simulink model "sldemo_tc_blocks"  (Simulink 7.6)
settings: Solver=FixedStepDiscrete  StartTime=0.0  StopTime=1  FixedStep=1  RelTol=1e-3
model workspace: external: MAT-File sldemo_tc_blocks_data.mat (data not in the file)
values from neighbouring files (symbols this model uses):
  TypeB_degC = TypeB_degC(1:2:end)    [sldemo_create_tc_blocks_data.m]    (also in sldemo_tc_blocks_data.mat = [0 2 4 6 8 10 12 14 16 18 20 22 ... (911 elements, 1x911)])
  TypeB_Volts = tcvoltage('B', TypeB_degC)    [sldemo_create_tc_blocks_data.m]    (also in sldemo_tc_blocks_data.mat = [0 -4.69410779782e-07 -8.91652511353e-07 -1.2667879384e-06 -)
  TypeE_degC = TypeE_degC(1:2:end)    [sldemo_create_tc_blocks_data.m]    (also in sldemo_tc_blocks_data.mat = [-270 -268 -266 -264 -262 -260 -258 -256 -254 -252 -250 -248)
  TypeE_Volts = tcvoltage('E', TypeE_degC)    [sldemo_create_tc_blocks_data.m]    (also in sldemo_tc_blocks_data.mat = [-0.00983495085619 -0.00983083480791 -0.00982483890705 -0.00)
  TypeJ_degC = TypeJ_degC(1:2:end)    [sldemo_create_tc_blocks_data.m]    (also in sldemo_tc_blocks_data.mat = [-210 -208 -206 -204 -202 -200 -198 -196 -194 -192 -190 -188)
  TypeJ_Volts = tcvoltage('J', TypeJ_degC)    [sldemo_create_tc_blocks_data.m]    (also in sldemo_tc_blocks_data.mat = [-0.0080953796493 -0.0080566195304 -0.00801673485998 -0.0079)
  TypeK_degC = TypeK_degC(1:2:end)    [sldemo_create_tc_blocks_data.m]    (also in sldemo_tc_blocks_data.mat = [-270 -268 -266 -264 -262 -260 -258 -256 -254 -252 -250 -248)
  TypeK_Volts = tcvoltage('K', TypeK_degC)    [sldemo_create_tc_blocks_data.m]    (also in sldemo_tc_blocks_data.mat = [-0.00645773795274 -0.00645592235046 -0.00645338583845 -0.00)
  TypeN_degC = TypeN_degC(1:2:end)    [sldemo_create_tc_blocks_data.m]    (also in sldemo_tc_blocks_data.mat = [-270 -268 -266 -264 -262 -260 -258 -256 -254 -252 -250 -248)
  TypeN_Volts = tcvoltage('N', TypeN_degC)    [sldemo_create_tc_blocks_data.m]    (also in sldemo_tc_blocks_data.mat = [-0.00434513544718 -0.00434422669637 -0.00434284037621 -0.00)
  TypeR_degC = TypeR_degC(1:2:end)    [sldemo_create_tc_blocks_data.m]    (also in sldemo_tc_blocks_data.mat = [-50 -48 -46 -44 -42 -40 -38 -36 -34 -32 -30 -28 ... (910 el)
  TypeR_Volts = tcvoltage('R', TypeR_degC)    [sldemo_create_tc_blocks_data.m]    (also in sldemo_tc_blocks_data.mat = [-0.000226465188174 -0.000218994213626 -0.00021137999827 -0.)
  TypeS_degC = TypeS_degC(1:2:end)    [sldemo_create_tc_blocks_data.m]    (also in sldemo_tc_blocks_data.mat = [-50 -48 -46 -44 -42 -40 -38 -36 -34 -32 -30 -28 ... (910 el)
  TypeS_Volts = tcvoltage('S', TypeS_degC)    [sldemo_create_tc_blocks_data.m]    (also in sldemo_tc_blocks_data.mat = [-0.000235555071493 -0.000227584395066 -0.000219482316956 -0)
  TypeT_degC = TypeT_degC(1:2:end)    [sldemo_create_tc_blocks_data.m]    (also in sldemo_tc_blocks_data.mat = [-270 -268 -266 -264 -262 -260 -258 -256 -254 -252 -250 -248)
  TypeT_Volts = tcvoltage('T', TypeT_degC)    [sldemo_create_tc_blocks_data.m]    (also in sldemo_tc_blocks_data.mat = [-0.00625750503786 -0.0062547569578 -0.00625068223974 -0.006)
Description:
  | ITS-90 Thermocouple Models
  | 
  | Full-Range 2 degrees Celsius Interpolated Thermocouple Tables created using
  | one ITS-90 Interpolating Polynomial and one inverse polynomial per junction type.
settings Model: Creator=The MathWorks Inc.  ExtModeAutoUpdateStatusClock=off  BufferReuse=off
settings OptimizationCC: BlockReduction=off  ConditionallyExecuteInputs=off  InlineInvariantSignals=on  OptimizeBlockIOStorage=off  BufferReuse=off  ExpressionFolding=off  LocalBlockOutputs=off  InitFltsAndDblsToZero=on  EfficientMapNaN2IntZero=off  BufferReusableBoundary=off
settings DebuggingCC: CheckExecutionContextPreStartOutputMsg=on  CheckExecutionContextRuntimeOutputMsg=on  SignalResolutionControl=TryResolveAllWithWarning  SolverPrmCheckMsg=none  MultiTaskDSMMsg=warning  MultiTaskCondExecSysMsg=none  UnconnectedInputMsg=none  UnconnectedOutputMsg=none  BusObjectLabelMismatch=none
settings RTWCC: IncludeERTFirstTime=on
settings CodeAppCC: CustomSymbolStrFcn=$F$N$M
settings GRTTargetCC: TargetFcnLib=ansi_tfl_tmw_new.mat

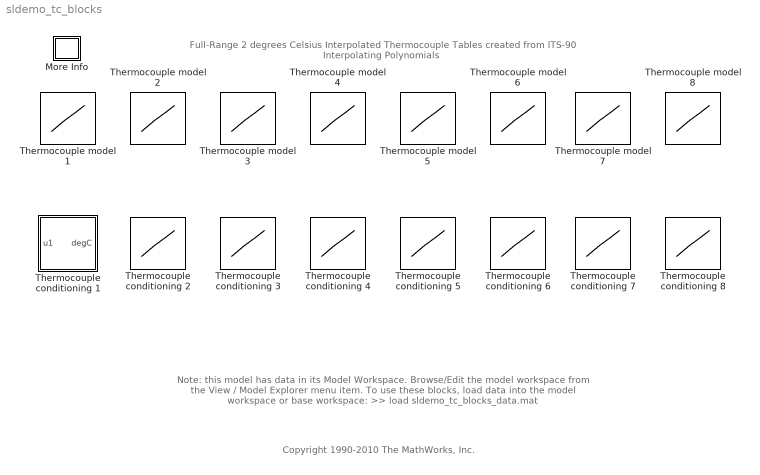
== system sldemo_tc_blocks ==
  note: Full-Range 2 degrees Celsius Interpolated Thermocouple Tables
      | created from ITS-90 Interpolating Polynomials
  note: Note: this model has data in its Model Workspace.
      | Browse/Edit the model workspace from the View / Model Explorer menu item.
      |
      | To use these blocks, load data into the model workspace or base workspace:
      | >> load sldemo_tc_blocks_data.mat
  note: Copyright 1990-2010 The MathWorks, Inc.
  More Info : Subsystem
      settings: OpenFcn=showdemo('sldemo_tc_script')
      mask Display: disp('?')
  Thermocouple conditioning 1 : Subsystem
      settings: AttributesFormatString=TypeB_Volts to\nTypeB_degC
      mask Display:
      | text(.15,.85,'1-D T(u)')
      | plot([0.3 0.3 0.95],[0.7 0.05 0.05])
      | plot([0.95 0.7515 0.554 0.4535 0.375 0.335 0.325],[0.7 0.6 0.5 0.4 0.3 0.2 0.05])
  Thermocouple conditioning 2 : Lookup_n-D  NumberOfTableDimensions=1  BreakpointsForDimension1=TypeE_Volts  BeginIndexSearchUsingPreviousIndexResult=on  Table=TypeE_degC  ActionForOutOfRangeInput=Warning  InputSameDT=on
      settings: AttributesFormatString=%<bp1> to\n%<tableData>
  Thermocouple conditioning 3 : Lookup_n-D  NumberOfTableDimensions=1  BreakpointsForDimension1=TypeJ_Volts  BeginIndexSearchUsingPreviousIndexResult=on  Table=TypeJ_degC  ActionForOutOfRangeInput=Warning  InputSameDT=on
      settings: AttributesFormatString=%<bp1> to\n%<tableData>
  Thermocouple conditioning 4 : Lookup_n-D  NumberOfTableDimensions=1  BreakpointsForDimension1=TypeK_Volts  BeginIndexSearchUsingPreviousIndexResult=on  Table=TypeK_degC  ActionForOutOfRangeInput=Warning  InputSameDT=on
      settings: AttributesFormatString=%<bp1> to\n%<tableData>
  Thermocouple conditioning 5 : Lookup_n-D  NumberOfTableDimensions=1  BreakpointsForDimension1=TypeN_Volts  BeginIndexSearchUsingPreviousIndexResult=on  Table=TypeN_degC  ActionForOutOfRangeInput=Warning  InputSameDT=on
      settings: AttributesFormatString=%<bp1> to\n%<tableData>
  Thermocouple conditioning 6 : Lookup_n-D  NumberOfTableDimensions=1  BreakpointsForDimension1=TypeR_Volts  BeginIndexSearchUsingPreviousIndexResult=on  Table=TypeR_degC  ActionForOutOfRangeInput=Warning  InputSameDT=on
      settings: AttributesFormatString=%<bp1> to\n%<tableData>
  Thermocouple conditioning 7 : Lookup_n-D  NumberOfTableDimensions=1  BreakpointsForDimension1=TypeS_Volts  BeginIndexSearchUsingPreviousIndexResult=on  Table=TypeS_degC  ActionForOutOfRangeInput=Warning  InputSameDT=on
      settings: AttributesFormatString=%<bp1> to\n%<tableData>
  Thermocouple conditioning 8 : Lookup_n-D  NumberOfTableDimensions=1  BreakpointsForDimension1=TypeT_Volts  BeginIndexSearchUsingPreviousIndexResult=on  Table=TypeT_degC  ActionForOutOfRangeInput=Warning  InputSameDT=on
      settings: AttributesFormatString=%<bp1> to\n%<tableData>
  Thermocouple model 1 : Lookup_n-D  NumberOfTableDimensions=1  BreakpointsForDimension1=TypeB_degC  BeginIndexSearchUsingPreviousIndexResult=on  Table=TypeB_Volts  ActionForOutOfRangeInput=Warning  InputSameDT=on
      settings: AttributesFormatString=%<bp1> to\n%<tableData>
  Thermocouple model 2 : Lookup_n-D  NumberOfTableDimensions=1  BreakpointsForDimension1=TypeE_degC  BeginIndexSearchUsingPreviousIndexResult=on  Table=TypeE_Volts  ActionForOutOfRangeInput=Warning  InputSameDT=on
      settings: AttributesFormatString=%<bp1> to\n%<tableData>
  Thermocouple model 3 : Lookup_n-D  NumberOfTableDimensions=1  BreakpointsForDimension1=TypeJ_degC  BeginIndexSearchUsingPreviousIndexResult=on  Table=TypeJ_Volts  ActionForOutOfRangeInput=Warning  InputSameDT=on
      settings: AttributesFormatString=%<bp1> to\n%<tableData>
  Thermocouple model 4 : Lookup_n-D  NumberOfTableDimensions=1  BreakpointsForDimension1=TypeK_degC  BeginIndexSearchUsingPreviousIndexResult=on  Table=TypeK_Volts  ActionForOutOfRangeInput=Warning  InputSameDT=on
      settings: AttributesFormatString=%<bp1> to\n%<tableData>
  Thermocouple model 5 : Lookup_n-D  NumberOfTableDimensions=1  BreakpointsForDimension1=TypeN_degC  BeginIndexSearchUsingPreviousIndexResult=on  Table=TypeN_Volts  ActionForOutOfRangeInput=Warning  InputSameDT=on
      settings: AttributesFormatString=%<bp1> to\n%<tableData>
  Thermocouple model 6 : Lookup_n-D  NumberOfTableDimensions=1  BreakpointsForDimension1=TypeR_degC  BeginIndexSearchUsingPreviousIndexResult=on  Table=TypeR_Volts  ActionForOutOfRangeInput=Warning  InputSameDT=on
      settings: AttributesFormatString=%<bp1> to\n%<tableData>
  Thermocouple model 7 : Lookup_n-D  NumberOfTableDimensions=1  BreakpointsForDimension1=TypeS_degC  BeginIndexSearchUsingPreviousIndexResult=on  Table=TypeS_Volts  ActionForOutOfRangeInput=Warning  InputSameDT=on
      settings: AttributesFormatString=%<bp1> to\n%<tableData>
  Thermocouple model 8 : Lookup_n-D  NumberOfTableDimensions=1  BreakpointsForDimension1=TypeT_degC  BeginIndexSearchUsingPreviousIndexResult=on  Table=TypeT_Volts  ActionForOutOfRangeInput=Warning  InputSameDT=on
      settings: AttributesFormatString=%<bp1> to\n%<tableData>

== system sldemo_tc_blocks/More Info ==

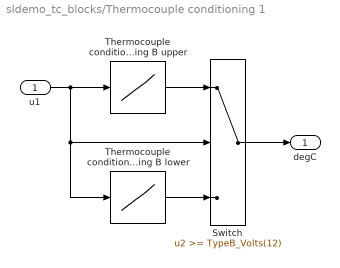
== system sldemo_tc_blocks/Thermocouple conditioning 1 ==
  u1 : Inport
  Switch : Switch  Threshold=TypeB_Volts(12)
  Thermocouple conditioning B lower : Lookup_n-D  NumberOfTableDimensions=1  BreakpointsForDimension1=TypeB_Volts(12:-1:1)  BeginIndexSearchUsingPreviousIndexResult=on  Table=TypeB_degC(12:-1:1)  ActionForOutOfRangeInput=Warning  InputSameDT=on
      settings: AttributesFormatString=%<bp1> to\n%<tableData>
  Thermocouple conditioning B upper : Lookup_n-D  NumberOfTableDimensions=1  BreakpointsForDimension1=TypeB_Volts(12:end)  BeginIndexSearchUsingPreviousIndexResult=on  Table=TypeB_degC(12:end)  ActionForOutOfRangeInput=Warning  InputSameDT=on
      settings: AttributesFormatString=%<bp1> to\n%<tableData>
  degC : Outport
  wires:
  Switch/1 -> degC/1
  Thermocouple conditioning B lower/1 -> Switch/3
  Thermocouple conditioning B upper/1 -> Switch/1
  u1/1 -> Switch/2, Thermocouple conditioning B lower/1, Thermocouple conditioning B upper/1
